simulink model "ABS_Model"  (R2020b)
settings: Solver=VariableStepAuto  StartTime=0.0  StopTime=10.0  RelTol=1e-3
PreLoadFcn:
  | abs_data;
model workspace (MAT data in the model file):
  Rr = 1.25
  g = 9.81
  m = 50
values from neighbouring files (symbols this model uses):
  mu = [0 .4 .8 .97 1.0 .98 .96 .94 .92 .9 .88 .855 .83 .81 .79 .77 .75 .73 .72 .71 .7]    [abs_data.m]
  slip = (0:.05:1.0)    [abs_data.m]
settings Model: Creator=ADMIN  LastModifiedBy=ADMIN

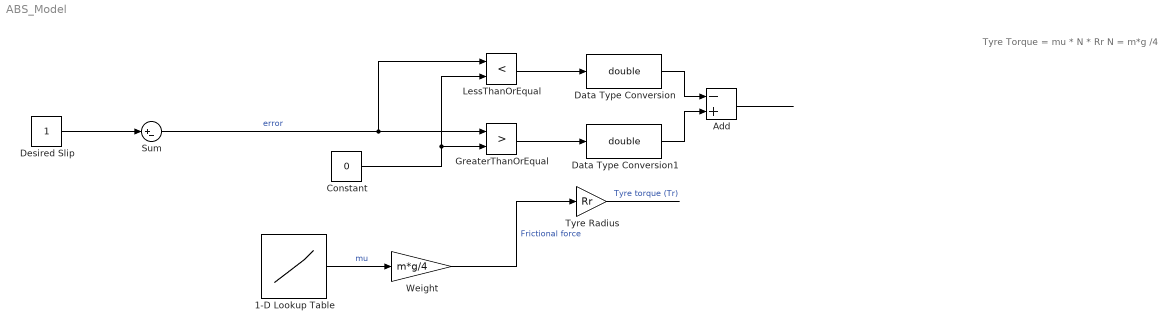
== system ABS_Model ==
  note: Tyre Torque = mu * N * Rr
      | N = m*g /4
  1-D Lookup Table : Lookup_n-D  NumberOfTableDimensions=1  BreakpointsForDimension1=slip  Table=mu  InternalRulePriority=Speed  RndMeth=Simplest  InputSameDT=on
  Add : Sum  Inputs=-+
  Constant : Constant  Value=0
  Data Type Conversion : DataTypeConversion  OutDataTypeStr=double
  Data Type Conversion1 : DataTypeConversion  OutDataTypeStr=double
  Desired Slip : Constant
  GreaterThanOrEqual : RelationalOperator  Operator=>  OutDataTypeStr=boolean  RndMeth=Simplest
  LessThanOrEqual : RelationalOperator  Operator=<  OutDataTypeStr=boolean  RndMeth=Simplest
  Sum : Sum  Inputs=|+-
  Tyre Radius : Gain  Gain=Rr
  Weight : Gain  Gain=m*g/4
  wires:
  ? -> Sum/2, 1-D Lookup Table/1
  1-D Lookup Table/1 -> Weight/1  "mu"
  Weight/1 -> Tyre Radius/1  "Frictional force"
  Tyre Radius/1 -> ?  "Tyre torque (Tr)"
  Desired Slip/1 -> Sum/1
  Sum/1 -> LessThanOrEqual/1, GreaterThanOrEqual/1  "error"
  Constant/1 -> LessThanOrEqual/2, GreaterThanOrEqual/2
  LessThanOrEqual/1 -> Data Type Conversion/1
  GreaterThanOrEqual/1 -> Data Type Conversion1/1
  Data Type Conversion/1 -> Add/1
  Data Type Conversion1/1 -> Add/2
  Add/1 -> ?
